simulink model "robotPrototype"  (R2021a)
settings: Solver=ode15s  StartTime=0.0  StopTime=simTime
model workspace: external: MAT-File (data not in the file)
values from neighbouring files (symbols this model uses):
  controlLim = [0.15 3 3]    [simulinkModelParam.mat]
  controlWeight = [0.75 0.6 0.5]    [simulinkModelParam.mat]
  delta = 0.3    [robotParameters.m]    (also in simulinkModelParam.mat = 0.25)
  deltaPlus = 0.20    (= 0.2)    [robotParameters.m]    (also in simulinkModelParam.mat = 0.15)
  den_CoP = [1 -1.84477840502 0.855986791935]    [simulinkModelParam.mat]
  den_zddot = [1 -1.92894226325 0.931381682127]    [simulinkModelParam.mat]
  f_0 = [1,1; deltaPlus-CoM_0(1), -(delta-deltaPlus+CoM_0(1))]\[m*9.81/2;0]    [robotParameters.m]
  f_sample = 500    [robotParameters.m]    (also in simulinkModelParam.mat = 1000)
  filterCoef = 50    [robotParameters.m]    (also in simulinkModelParam.mat = 1000)
  foot_x = delta    (= 0.3)    [robotParameters.m]    (also in simulinkModelParam.mat = 0.25)
  foot_y = delta/3    (= 0.1)    [robotParameters.m]    (also in simulinkModelParam.mat = 0.0833333333333)
  foot_z = 0.03    [robotParameters.m]    (also in simulinkModelParam.mat = 0.02)
  kd_ank = 0    [robotParameters.m]    (also in simulinkModelParam.mat)
  kd_hip = 250    [robotParameters.m]    (also in simulinkModelParam.mat = 12)
  kd_knee1 = 0.02    [robotParameters.m]    (also in simulinkModelParam.mat = 0)
  kd_knee2 = 500    [robotParameters.m]    (also in simulinkModelParam.mat = 150)
  ki_ank = 1800    [robotParameters.m]    (also in simulinkModelParam.mat = 500)
  ki_hip = 0    [robotParameters.m]    (also in simulinkModelParam.mat)
  ki_knee1 = 0    [robotParameters.m]    (also in simulinkModelParam.mat = 0.5)
  ki_knee2 = 0    [robotParameters.m]    (also in simulinkModelParam.mat)
  kp_ank = 375    [robotParameters.m]    (also in simulinkModelParam.mat = 325)
  kp_hip = 500    [robotParameters.m]    (also in simulinkModelParam.mat = 25)
  kp_knee1 = 8    [robotParameters.m]    (also in simulinkModelParam.mat = 3)
  kp_knee2 = 1000    [robotParameters.m]    (also in simulinkModelParam.mat = 300)
  L = 0.94*2*legLength    (= 0.7896)    [robotParameters.m]    (also in simulinkModelParam.mat = 0.72)
  legLength = param(1)    [forwardKin.m]    (also in robotParameters.m = 0.42; simulinkModelParam.mat = 0.4)
  legWidth = 0.08    [robotParameters.m]    (also in simulinkModelParam.mat = 0.05)
  limbThickness = 0.05    [robotParameters.m]    (also in simulinkModelParam.mat = 0.025)
  m = param(3)    [forwardKin.m]    (also in robotParameters.m = 70; simulinkModelParam.mat = 25)
  modelProperties = [25 0.5781 0.72]    [simulinkModelParam.mat]
  N = length(theta)    [robotParameters.m]
  num_CoP = [0.00280209672777 0.00560419345555 0.00280209672777]    [simulinkModelParam.mat]
  num_zddot = [0.000609854718717 0.00121970943743 0.000609854718717]    [simulinkModelParam.mat]
  p = 28    [simulinkModelParam.mat]
  pushDur = 0.1    [compareReducedOrderModels.m]    (also in simulinkModelParam.mat; startUpBalanceRobot.m)
  pushForce = pushForce - 2*pushStep    (= 0)    [compareReducedOrderModels.m]    (also in startUpBalanceRobot.m = 494)
  pushOnset = 0.2    [compareReducedOrderModels.m]    (also in simulinkModelParam.mat; startUpBalanceRobot.m)
  segmentMass = struct('torso',0.681, 'thigh', 0.2, 'shank', 0.09, 'foot', 0.029)    [robotParameters.m]
  stateLim = [0.15 1.57079632679 0.8 0.55 1.622 0.3]    [simulinkModelParam.mat]
  stateWeight = [3 0.5 0.3 9 0.25 0.09]    [simulinkModelParam.mat]
  support_x = 2.5    [robotParameters.m]    (also in simulinkModelParam.mat)
  support_y = 2.5    [robotParameters.m]    (also in simulinkModelParam.mat)
  support_z = 0.1    [robotParameters.m]    (also in simulinkModelParam.mat)
  torsoCoM = param(2)    [forwardKin.m]    (also in robotParameters.m = 0.235; simulinkModelParam.mat = 0.1875)
  torsoLength = 0.47    [robotParameters.m]    (also in simulinkModelParam.mat = 0.25)
  zmax = (2*legLength)*sin(acos(0.2/(2*legLength)))+ankleOffset    [robotParameters.m]    (also in simulinkModelParam.mat = 0.8)
  zmin = 0.6+ ankleOffset    (= 0.67)    [robotParameters.m]    (also in simulinkModelParam.mat = 0.6)
undefined symbols (not defined in the file or in its folder): controlRateWeight, den_qdot, nlobjLIP, num_qdot, X, Y, Z
libraries: sm_lib x27, nesl_utility x19, pid_lib x16, robotmaniplib x16, simulink_extras x16, mpclib x4, Contact_Forces_Lib x4, simulink x2
(part 1 of 3)
settings Model: SimulationMode=accelerator  OrderedModelArguments=off  Creator=tomhu  LastModifiedBy=tomhu
settings SimscapeCC: SimscapeNormalizeSystem=off
settings DiagnosticsConfigSet: SimMechanicsRigidlyBoundBlock=warning
settings ExplorerConfigSet: SimMechanicsOpenEditorOnUpdate=off

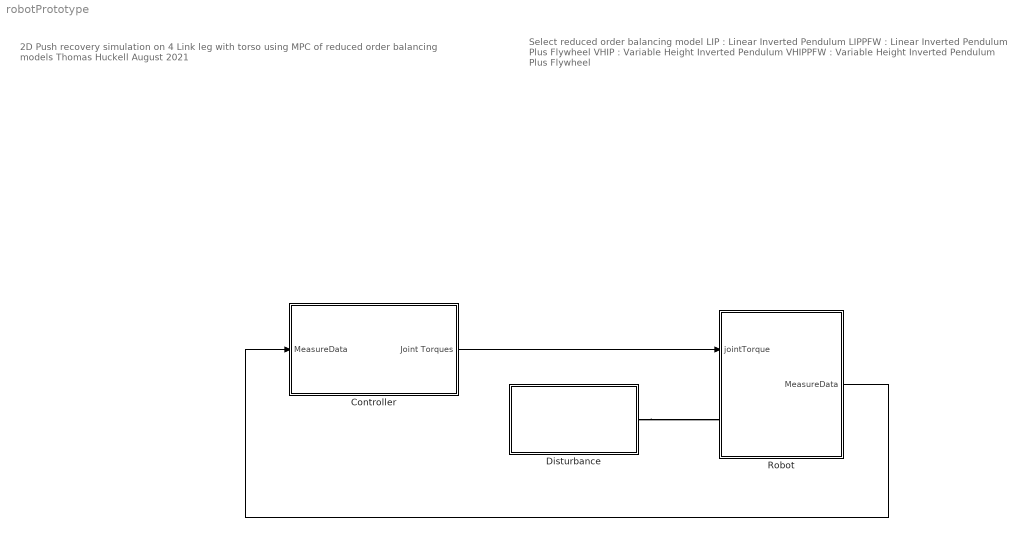
== system robotPrototype ==
  note: Select reduced order balancing model
      | LIP : Linear Inverted Pendulum
      | LIPPFW : Linear Inverted Pendulum Plus Flywheel
      | VHIP : Variable Height Inverted Pendulum
      | VHIPPFW : Variable Height Inverted Pendulum Plus Flywheel
  note: 2D Push recovery simulation on 4 Link leg with torso using MPC of reduced order balancing models
      |
      | Thomas Huckell
      |
      | August 2021
  Controller : Subsystem
  Disturbance : Subsystem  mask{M=pushForce, pushDur=pushDur, Ts=pushOnset}
      mask prompts: M "Push Force [N]"; pushDur "Push Duration [s]"; Ts "Push Onset [s]"
  Robot : Subsystem
      mask Display: image('C:\Users\tomhu\OneDrive - Queen''s University\MASc\Research\Robot\Model\Figures\RobotConfigure.PNG'); % Use "Edit Image" on toolstrip to change.
  wires:
  Controller/1(Joint Torques) -> Robot/1(jointTorque)
  Robot/1(MeasureData) -> Controller/1(MeasureData)
  connections:
  Disturbance/RConn1 -- Robot/LConn1

== system robotPrototype/Controller ==
  MeasureData : Inport
  Bus Creator : BusCreator  Inputs=3
  Bus Selector : BusSelector  OutputSignals=state
  Bus Selector1 : BusSelector  OutputSignals=ankle,knee,hip
  MPC : Subsystem  Variant=on
  Saturation1 : Saturate  UpperLimit=500  LowerLimit=-500  LinearizeAsGain=off
  Saturation2 : Saturate  UpperLimit=500  LowerLimit=-500  LinearizeAsGain=off
  Saturation3 : Saturate  UpperLimit=500  LowerLimit=-500  LinearizeAsGain=off
  To Workspace : ToWorkspace  VariableName=jointTorques  SaveFormat=Timeseries  SampleTime=-1
  To Workspace1 : ToWorkspace  VariableName=mpcControl  SaveFormat=Timeseries  SampleTime=-1
  Variant Subsystem : Subsystem  Variant=on
  Joint Torques : Outport
  wires:
  Bus Selector/1 -> MPC/1(X)  "<state>"
  MeasureData/1 -> Variant Subsystem/2(measureData), Bus Selector/1
  MPC/1(mv) -> To Workspace1/1, Variant Subsystem/1(mv)
  Variant Subsystem/1(jointTorque) -> Bus Selector1/1
  Bus Creator/1 -> To Workspace/1, Joint Torques/1
  Saturation2/1 -> Bus Creator/1  "ankle"
  Saturation1/1 -> Bus Creator/2  "knee"
  Saturation3/1 -> Bus Creator/3  "hip"
  Bus Selector1/1 -> Saturation2/1  "<ankle>"
  Bus Selector1/2 -> Saturation1/1  "<knee>"
  Bus Selector1/3 -> Saturation3/1  "<hip>"

== system robotPrototype/Disturbance ==
  Add : Sum
  External Force and Torque : sm_lib/Forces and Torques/External Force and Torque  ForceResolutionFrame=AttachedFrame  EnableForceX=on  EnableForceY=off  EnableForceZ=off  EnableForce=off  TorqueResolutionFrame=AttachedFrame  EnableTorqueX=off  EnableTorqueY=off  EnableTorqueZ=off  EnableTorque=off
  Simulink-PS Converter4 : nesl_utility/Simulink-PS Converter  PhysicalDomain=network_engine_domain  SubClassName=ps_input  LeftPortType=input  RightPortType=output  PseudoPeriodic=off  Frequencies=[]  NoiseDistribution=none  NoiseParameters=[]  Unit=1  AffineConversion=off  FilteringAndDerivatives=provide  SimscapeFilterOrder=1  InputFilterTimeConstant=0.001  UdotUserProvided=0
      settings: SourceProductBaseCode=PW,SS
  Step : Step  Time=Ts  After=M  SampleTime=0
  Step1 : Step  Time=Ts+pushDur  After=-M  SampleTime=0
  Push Disturbance : PMIOPort  Side=Right
  wires:
  Add/1 -> Simulink-PS Converter4/1
  Step/1 -> Add/1
  Step1/1 -> Add/2
  connections:
  Simulink-PS Converter4/RConn1 -- External Force and Torque/LConn1
  External Force and Torque/RConn1 -- Push Disturbance/RConn1

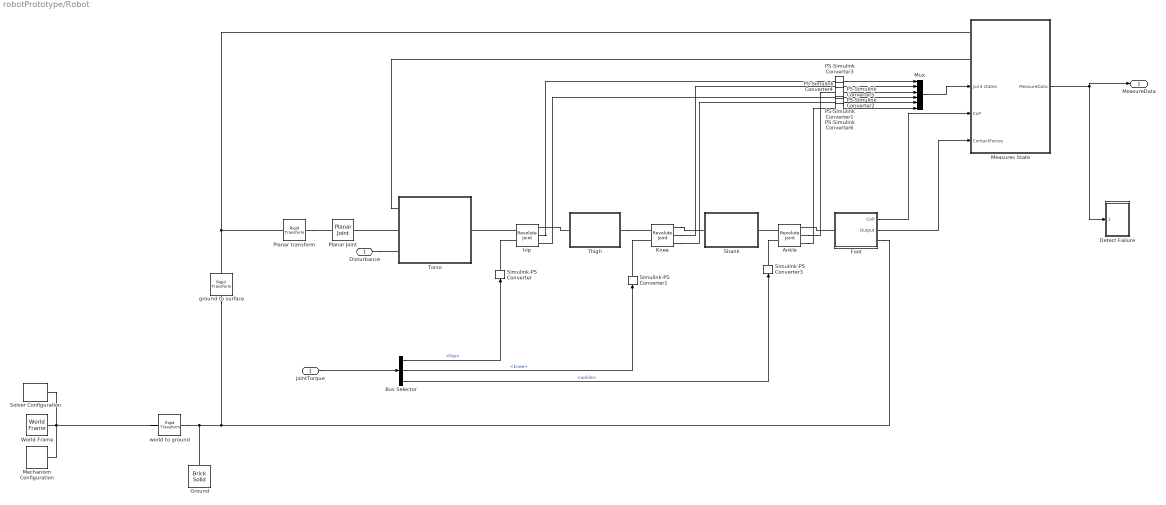
== system robotPrototype/Robot ==
  jointTorque : Inport
  Ankle : sm_lib/Joints/Revolute Joint  JointMode=Normal  SenseConstraintForce=off  SenseConstraintForceX=off  SenseConstraintForceY=off  SenseConstraintForceZ=off  SenseConstraintTorque=off  SenseConstraintTorqueX=off  SenseConstraintTorqueY=off  SenseConstraintTorqueZ=off  SenseTotalForce=off  SenseTotalForceX=off  SenseTotalForceY=off  SenseTotalForceZ=off  SenseTotalTorque=off  SenseTotalTorqueX=off  SenseTotalTorqueY=off  SenseTotalTorqueZ=off  CompositeWrenchDir=FollowerOnBase  CompositeWrenchFrame=BaseFrame  EquilibriumPosition=0  EquilibriumPositionUnits=deg  SpringStiffness=0  SpringStiffnessUnits=N*m/deg  DampingCoefficient=0.001  DampingCoefficientUnits=N*m/(deg/s)  TorqueActuationMode=InputTorque  MotionActuationMode=ComputedMotion  SensePosition=on  SenseVelocity=on  SenseAcceleration=off  SenseTorqueForce=off  SenseLowerLimitTorqueForce=off  SenseUpperLimitTorqueForce=off  LowerLimitSpecify=on  LowerLimitBound=-90  LowerLimitBoundUnits=deg  LowerLimitStiffness=1e4  LowerLimitStiffnessUnits=N*m/deg  LowerLimitDamping=10  LowerLimitDampingUnits=N*m/(deg/s)  LowerLimitTransitionRegionWidth=0.1  LowerLimitTransitionRegionWidthUnits=deg  UpperLimitSpecify=on  UpperLimitBound=90  UpperLimitBoundUnits=deg  UpperLimitStiffness=1e4  UpperLimitStiffnessUnits=N*m/deg  UpperLimitDamping=10  UpperLimitDampingUnits=N*m/(deg/s)  UpperLimitTransitionRegionWidth=0.1  UpperLimitTransitionRegionWidthUnits=deg  PositionTargetSpecify=on  PositionTargetPriority=High  PositionTargetValue=t3_0  PositionTargetValueUnits=rad  VelocityTargetSpecify=off  VelocityTargetPriority=High  VelocityTargetValue=0  VelocityTargetValueUnits=deg/s
  Bus Selector : BusSelector  OutputSignals=hip,knee,ankle
  Detect Failure : Subsystem
  Foot : Subsystem
  Ground : sm_lib/Body Elements/Brick Solid  GraphicAmbientColor=[0.15 0.15 0.15 1.0]  BasedOnType=Density  BrickDimensions=[support_x, support_y, support_z]  BrickDimensionUnits=m  CenterOfMass=[0 0 0]  CenterOfMassUnits=m  GraphicDiffuseColor=[0.0 0.4 0.2]  Density=1000  DensityUnits=kg/m^3  DoExposeReferenceFrame=on  GraphicEmissiveColor=[0.0 0.0 0.0 1.0]  ExportEntireGeometry=off  SerializedFrames=<Frames/>  MarkerShape=Sphere  MarkerSize=10  GraphicType=FromGeometry  InertiaType=CalculateFromGeometry  Mass=1  MassUnits=kg  MomentsOfInertia=[1 1 1]  MomentsOfInertiaUnits=kg*m^2  GraphicOpacity=0.3  ProductsOfInertia=[0 0 0]  ProductsOfInertiaUnits=kg*m^2  GraphicShininess=75  GraphicSpecularColor=[0.5 0.5 0.5 1.0]  GraphicVisPropType=SimpleVisualProperties
  Knee : sm_lib/Joints/Revolute Joint  JointMode=Normal  SenseConstraintForce=off  SenseConstraintForceX=off  SenseConstraintForceY=off  SenseConstraintForceZ=off  SenseConstraintTorque=off  SenseConstraintTorqueX=off  SenseConstraintTorqueY=off  SenseConstraintTorqueZ=off  SenseTotalForce=off  SenseTotalForceX=off  SenseTotalForceY=off  SenseTotalForceZ=off  SenseTotalTorque=off  SenseTotalTorqueX=off  SenseTotalTorqueY=off  SenseTotalTorqueZ=off  CompositeWrenchDir=FollowerOnBase  CompositeWrenchFrame=BaseFrame  EquilibriumPosition=0  EquilibriumPositionUnits=deg  SpringStiffness=0  SpringStiffnessUnits=N*m/deg  DampingCoefficient=0.001  DampingCoefficientUnits=N*m/(deg/s)  TorqueActuationMode=InputTorque  MotionActuationMode=ComputedMotion  SensePosition=on  SenseVelocity=on  SenseAcceleration=off  SenseTorqueForce=off  SenseLowerLimitTorqueForce=off  SenseUpperLimitTorqueForce=off  LowerLimitSpecify=on  LowerLimitBound=-90  LowerLimitBoundUnits=deg  LowerLimitStiffness=1e5  LowerLimitStiffnessUnits=N*m/deg  LowerLimitDamping=10  LowerLimitDampingUnits=N*m/(deg/s)  LowerLimitTransitionRegionWidth=3  LowerLimitTransitionRegionWidthUnits=deg  UpperLimitSpecify=on  UpperLimitBound=0  UpperLimitBoundUnits=deg  UpperLimitStiffness=1e4  UpperLimitStiffnessUnits=N*m/deg  UpperLimitDamping=10  UpperLimitDampingUnits=N*m/(deg/s)  UpperLimitTransitionRegionWidth=2  UpperLimitTransitionRegionWidthUnits=deg  PositionTargetSpecify=on  PositionTargetPriority=High  PositionTargetValue=t2_0  PositionTargetValueUnits=rad  VelocityTargetSpecify=off  VelocityTargetPriority=High  VelocityTargetValue=0  VelocityTargetValueUnits=deg/s
  Measures State : Subsystem
      settings: PortSchema="{\"entries\":[{\"content\":{\"sides\":[{\"content\":{\"connectorIds\":[\"LConn1\",\"LConn2\",\"In1\",\"In2\",\"In3\"]},\"type\":\"ConnectorPlacement.EquallySpacedRectSide\",\"uuid\":\"491601c2-282d-472b-a160-449a44ca8289\"},{\"content\":{\"connectorIds\":[\"Out1\"],\"side\":\"RIGHT\"},\"type\":\"ConnectorPlacement.EquallySpacedRectSide\",\"uuid\":\"5be6c390-8aea-4246-9e11-8b08edaa1b58\"},{\"content\":{\"connectorIds\":[],\"side\":\"TOP\"},\"type\":\"ConnectorPlacement.EquallySpacedRectSide\",\"uuid\":\"78d05e4f-efd7-46b6-ad15-3acf80423762\"}]},\"type\":\"ConnectorPlacement.EquallySpacedConnector\",\"uuid\":\"639014c9-32ba-4b2e-824a-b04e55a10a1e\"}],\"packageUris\":[\"http://schema.mathworks.com/mf0/Connector/R2020b\"],\"version\":\"1.0\"}"
  Mechanism Configuration : sm_lib/Utilities/Mechanism Configuration  UniformGravity=Constant  GravityVector=[0 0 -9.80665]  GravityVectorUnits=m/s^2  GravityUnits=m/s^2  LinearizationDelta=0.001  JointModeTransitionNonlinearIterations=2
  Mux : Mux  Inputs=6
  PS-Simulink Converter1 : nesl_utility/PS-Simulink Converter  PhysicalDomain=network_engine_domain  SubClassName=ps_output  LeftPortType=input  RightPortType=output  PseudoPeriodic=off  Frequencies=[]  Unit=rad/s  AffineConversion=off
      settings: SourceProductBaseCode=PW,SS
  PS-Simulink Converter2 : nesl_utility/PS-Simulink Converter  PhysicalDomain=network_engine_domain  SubClassName=ps_output  LeftPortType=input  RightPortType=output  PseudoPeriodic=off  Frequencies=[]  Unit=rad/s  AffineConversion=off
      settings: SourceProductBaseCode=PW,SS
  PS-Simulink Converter3 : nesl_utility/PS-Simulink Converter  PhysicalDomain=network_engine_domain  SubClassName=ps_output  LeftPortType=input  RightPortType=output  PseudoPeriodic=off  Frequencies=[]  Unit=rad  AffineConversion=off
      settings: SourceProductBaseCode=PW,SS
  PS-Simulink Converter4 : nesl_utility/PS-Simulink Converter  PhysicalDomain=network_engine_domain  SubClassName=ps_output  LeftPortType=input  RightPortType=output  PseudoPeriodic=off  Frequencies=[]  Unit=rad  AffineConversion=off
      settings: SourceProductBaseCode=PW,SS
  PS-Simulink Converter5 : nesl_utility/PS-Simulink Converter  PhysicalDomain=network_engine_domain  SubClassName=ps_output  LeftPortType=input  RightPortType=output  PseudoPeriodic=off  Frequencies=[]  Unit=rad  AffineConversion=off
      settings: SourceProductBaseCode=PW,SS
  PS-Simulink Converter6 : nesl_utility/PS-Simulink Converter  PhysicalDomain=network_engine_domain  SubClassName=ps_output  LeftPortType=input  RightPortType=output  PseudoPeriodic=off  Frequencies=[]  Unit=rad/s  AffineConversion=off
      settings: SourceProductBaseCode=PW,SS
  Planar Joint : sm_lib/Joints/Planar Joint  JointMode=Normal  SenseConstraintForce=off  SenseConstraintForceX=off  SenseConstraintForceY=off  SenseConstraintForceZ=off  SenseConstraintTorque=off  SenseConstraintTorqueX=off  SenseConstraintTorqueY=off  SenseConstraintTorqueZ=off  SenseTotalForce=off  SenseTotalForceX=off  SenseTotalForceY=off  SenseTotalForceZ=off  SenseTotalTorque=off  SenseTotalTorqueX=off  SenseTotalTorqueY=off  SenseTotalTorqueZ=off  CompositeWrenchDir=FollowerOnBase  CompositeWrenchFrame=BaseFrame  PxEquilibriumPosition=0  PxEquilibriumPositionUnits=m  PxSpringStiffness=0  PxSpringStiffnessUnits=N/m  PxDampingCoefficient=0  PxDampingCoefficientUnits=N/(m/s)  PxTorqueActuationMode=NoTorque  PxMotionActuationMode=ComputedMotion  PxSensePosition=off  PxSenseVelocity=off  PxSenseAcceleration=off  PxSenseTorqueForce=off  PxSenseLowerLimitTorqueForce=off  PxSenseUpperLimitTorqueForce=off  PxLowerLimitSpecify=off  PxLowerLimitBound=-1  PxLowerLimitBoundUnits=m  PxLowerLimitStiffness=1e6  PxLowerLimitStiffnessUnits=N/m  PxLowerLimitDamping=1e3  PxLowerLimitDampingUnits=N/(m/s)  PxLowerLimitTransitionRegionWidth=1e-4  PxLowerLimitTransitionRegionWidthUnits=m  PxUpperLimitSpecify=off  PxUpperLimitBound=1  PxUpperLimitBoundUnits=m  PxUpperLimitStiffness=1e6  PxUpperLimitStiffnessUnits=N/m  PxUpperLimitDamping=1e3  PxUpperLimitDampingUnits=N/(m/s)  PxUpperLimitTransitionRegionWidth=1e-4  PxUpperLimitTransitionRegionWidthUnits=m  PxPositionTargetSpecify=off  PxPositionTargetPriority=High  PxPositionTargetValue=0  PxPositionTargetValueUnits=m  PxVelocityTargetSpecify=off  PxVelocityTargetPriority=High  PxVelocityTargetValue=0  PxVelocityTargetValueUnits=m/s  PyEquilibriumPosition=0  PyEquilibriumPositionUnits=m  PySpringStiffness=0  PySpringStiffnessUnits=N/m  PyDampingCoefficient=0  PyDampingCoefficientUnits=N/(m/s)  PyTorqueActuationMode=NoTorque  PyMotionActuationMode=ComputedMotion  PySensePosition=off  PySenseVelocity=off  PySenseAcceleration=off  PySenseTorqueForce=off  PySenseLowerLimitTorqueForce=off  PySenseUpperLimitTorqueForce=off  PyLowerLimitSpecify=off  PyLowerLimitBound=-1  PyLowerLimitBoundUnits=m  PyLowerLimitStiffness=1e6  PyLowerLimitStiffnessUnits=N/m  PyLowerLimitDamping=1e3  PyLowerLimitDampingUnits=N/(m/s)  PyLowerLimitTransitionRegionWidth=1e-4  PyLowerLimitTransitionRegionWidthUnits=m  PyUpperLimitSpecify=off  PyUpperLimitBound=1  PyUpperLimitBoundUnits=m  PyUpperLimitStiffness=1e6  PyUpperLimitStiffnessUnits=N/m  PyUpperLimitDamping=1e3  PyUpperLimitDampingUnits=N/(m/s)  PyUpperLimitTransitionRegionWidth=1e-4  PyUpperLimitTransitionRegionWidthUnits=m  PyPositionTargetSpecify=on  PyPositionTargetPriority=High  PyPositionTargetValue="L+torsoLength -  4.4100e-04"  PyPositionTargetValueUnits=m  PyVelocityTargetSpecify=off  PyVelocityTargetPriority=High  PyVelocityTargetValue=0  PyVelocityTargetValueUnits=m/s  RzEquilibriumPosition=0  RzEquilibriumPositionUnits=deg  RzSpringStiffness=0  RzSpringStiffnessUnits=N*m/deg  RzDampingCoefficient=0  RzDampingCoefficientUnits=N*m/(deg/s)  RzTorqueActuationMode=NoTorque  RzMotionActuationMode=ComputedMotion  RzSensePosition=off  RzSenseVelocity=off  RzSenseAcceleration=off  RzSenseTorqueForce=off  RzSenseLowerLimitTorqueForce=off  RzSenseUpperLimitTorqueForce=off  RzLowerLimitSpecify=off  RzLowerLimitBound=-90  RzLowerLimitBoundUnits=deg  RzLowerLimitStiffness=1e4  RzLowerLimitStiffnessUnits=N*m/deg  RzLowerLimitDamping=10  RzLowerLimitDampingUnits=N*m/(deg/s)  RzLowerLimitTransitionRegionWidth=0.1  RzLowerLimitTransitionRegionWidthUnits=deg  RzUpperLimitSpecify=off  RzUpperLimitBound=90  RzUpperLimitBoundUnits=deg  RzUpperLimitStiffness=1e4  RzUpperLimitStiffnessUnits=N*m/deg  RzUpperLimitDamping=10  RzUpperLimitDampingUnits=N*m/(deg/s)  RzUpperLimitTransitionRegionWidth=0.1  RzUpperLimitTransitionRegionWidthUnits=deg  RzPositionTargetSpecify=off  RzPositionTargetPriority=High  RzPositionTargetValue=0  RzPositionTargetValueUnits=deg  RzVelocityTargetSpecify=off  RzVelocityTargetPriority=High  RzVelocityTargetValue=0  RzVelocityTargetValueUnits=deg/s
  Planer transform : sm_lib/Frames and Transforms/Rigid Transform  TranslationMethod=None  TranslationStandardOffset=0  TranslationLengthUnit=m  TranslationStandardAxis=+Z  TranslationCartesianOffset=[0 0 0]  TranslationROffset=0  TranslationROffsetUnits=m  TranslationZOffset=0  TranslationZOffsetUnits=m  TranslationThetaOffset=0  TranslationThetaOffsetUnits=deg  RotationMethod=StandardAxis  RotationAngleUnits=deg  RotationStandardAxis=+X  RotationAngle=90  RotationArbitraryAxis=[0 0 1]  FollAlignAxisA=+X  BaseAlignAxisA=+Y  FollAlignAxisB=+Y  BaseAlignAxisB=+Z  RotationSequenceAxes=FollowerAxes  RotationSequence=XYX  RotationSequenceAngles=[0 0 0]  RotationSequenceAnglesUnits=deg  RotationMatrix=[1 0 0; 0 1 0; 0 0 1]
  Shank : Subsystem
  Simulink-PS Converter : nesl_utility/Simulink-PS Converter  PhysicalDomain=network_engine_domain  SubClassName=ps_input  LeftPortType=input  RightPortType=output  PseudoPeriodic=off  Frequencies=[]  NoiseDistribution=none  NoiseParameters=[]  Unit=1  AffineConversion=off  FilteringAndDerivatives=provide  SimscapeFilterOrder=1  InputFilterTimeConstant=0.001  UdotUserProvided=0
      settings: SourceProductBaseCode=PW,SS
  Simulink-PS Converter1 : nesl_utility/Simulink-PS Converter  PhysicalDomain=network_engine_domain  SubClassName=ps_input  LeftPortType=input  RightPortType=output  PseudoPeriodic=off  Frequencies=[]  NoiseDistribution=none  NoiseParameters=[]  Unit=1  AffineConversion=off  FilteringAndDerivatives=provide  SimscapeFilterOrder=1  InputFilterTimeConstant=0.001  UdotUserProvided=0
      settings: SourceProductBaseCode=PW,SS
  Simulink-PS Converter3 : nesl_utility/Simulink-PS Converter  PhysicalDomain=network_engine_domain  SubClassName=ps_input  LeftPortType=input  RightPortType=output  PseudoPeriodic=off  Frequencies=[]  NoiseDistribution=none  NoiseParameters=[]  Unit=1  AffineConversion=off  FilteringAndDerivatives=provide  SimscapeFilterOrder=1  InputFilterTimeConstant=0.001  UdotUserProvided=0
      settings: SourceProductBaseCode=PW,SS
  Solver Configuration : nesl_utility/Solver Configuration  PhysicalDomain=network_engine_domain  SubClassName=solver  LeftPortType=input  RightPortType=generic  Tones=[]  Harmonics=[]  SimulateNoise=off  Profile=off  UseLocalSampling=off  EnableSwitchedLinearOptims=on  FrequencyDomain=off  UseCCode=off  RelTol=0.001  AbsTol=1e-06  MinStep=1e-09  ToWorkspace=off  RevertToSquareIcSolve=off  NumHomotopyIterations=100  PhasorMode=off  PhasorModeNumHarmonics=1  DoDC=off  ResidualTolerance=1e-09  UseLocalSolver=off  LocalSolverChoice=NE_TRAPEZOIDAL_ADVANCER  LocalSolverSampleTime=0.001  DoFixedCost=off  MaxNonlinIter=3  MaxModeIter=2  ComputeImpulses=off  ImpulseIterations=2  LinearAlgebra=Sparse  EquationFormulation=NE_TIME_EF  DelaysMemoryBudget=1024  AutomaticFiltering=on  FilteringTimeConstant=0.001  PartitionStorageMethod=AS_NEEDED  PartitionMemoryBudget=1024  PartitionMethod=ROBUST
      settings: SourceProductBaseCode=PW,SS
  Thigh : Subsystem
  Torso : Subsystem
  World Frame : sm_lib/Frames and Transforms/World Frame
  ground to surface : sm_lib/Frames and Transforms/Rigid Transform  TranslationMethod=StandardAxis  TranslationStandardOffset=1/2*support_z  TranslationLengthUnit=m  TranslationStandardAxis=+Z  TranslationCartesianOffset=[0 0 0]  TranslationROffset=0  TranslationROffsetUnits=m  TranslationZOffset=0  TranslationZOffsetUnits=m  TranslationThetaOffset=0  TranslationThetaOffsetUnits=deg  RotationMethod=None  RotationAngleUnits=deg  RotationStandardAxis=+Z  RotationAngle=0.0  RotationArbitraryAxis=[0 0 1]  FollAlignAxisA=+X  BaseAlignAxisA=+Y  FollAlignAxisB=+Y  BaseAlignAxisB=+Z  RotationSequenceAxes=FollowerAxes  RotationSequence=XYX  RotationSequenceAngles=[0 0 0]  RotationSequenceAnglesUnits=deg  RotationMatrix=[1 0 0; 0 1 0; 0 0 1]
  hip : sm_lib/Joints/Revolute Joint  JointMode=Normal  SenseConstraintForce=off  SenseConstraintForceX=off  SenseConstraintForceY=off  SenseConstraintForceZ=off  SenseConstraintTorque=off  SenseConstraintTorqueX=off  SenseConstraintTorqueY=off  SenseConstraintTorqueZ=off  SenseTotalForce=off  SenseTotalForceX=off  SenseTotalForceY=off  SenseTotalForceZ=off  SenseTotalTorque=off  SenseTotalTorqueX=off  SenseTotalTorqueY=off  SenseTotalTorqueZ=off  CompositeWrenchDir=FollowerOnBase  CompositeWrenchFrame=BaseFrame  EquilibriumPosition=0  EquilibriumPositionUnits=deg  SpringStiffness=0  SpringStiffnessUnits=N*m/deg  DampingCoefficient=0.001  DampingCoefficientUnits=N*m/(deg/s)  TorqueActuationMode=InputTorque  MotionActuationMode=ComputedMotion  SensePosition=on  SenseVelocity=on  SenseAcceleration=off  SenseTorqueForce=off  SenseLowerLimitTorqueForce=off  SenseUpperLimitTorqueForce=off  LowerLimitSpecify=on  LowerLimitBound=-120  LowerLimitBoundUnits=deg  LowerLimitStiffness=1e4  LowerLimitStiffnessUnits=N*m/deg  LowerLimitDamping=10  LowerLimitDampingUnits=N*m/(deg/s)  LowerLimitTransitionRegionWidth=5  LowerLimitTransitionRegionWidthUnits=deg  UpperLimitSpecify=on  UpperLimitBound=120  UpperLimitBoundUnits=deg  UpperLimitStiffness=1e4  UpperLimitStiffnessUnits=N*m/deg  UpperLimitDamping=10  UpperLimitDampingUnits=N*m/(deg/s)  UpperLimitTransitionRegionWidth=5  UpperLimitTransitionRegionWidthUnits=deg  PositionTargetSpecify=on  PositionTargetPriority=High  PositionTargetValue=t1_0  PositionTargetValueUnits=rad  VelocityTargetSpecify=off  VelocityTargetPriority=High  VelocityTargetValue=0  VelocityTargetValueUnits=deg/s
  world to ground : sm_lib/Frames and Transforms/Rigid Transform  TranslationMethod=Cartesian  TranslationStandardOffset=0  TranslationLengthUnit=m  TranslationStandardAxis=+Z  TranslationCartesianOffset=[0 0 0]  TranslationROffset=0  TranslationROffsetUnits=m  TranslationZOffset=0  TranslationZOffsetUnits=m  TranslationThetaOffset=0  TranslationThetaOffsetUnits=deg  RotationMethod=None  RotationAngleUnits=deg  RotationStandardAxis=+Z  RotationAngle=0.0  RotationArbitraryAxis=[0 0 1]  FollAlignAxisA=+X  BaseAlignAxisA=+Y  FollAlignAxisB=+Y  BaseAlignAxisB=+Z  RotationSequenceAxes=FollowerAxes  RotationSequence=XYX  RotationSequenceAngles=[0 0 0]  RotationSequenceAnglesUnits=deg  RotationMatrix=[1 0 0; 0 1 0; 0 0 1]
  Disturbance : PMIOPort  Side=Left
  MeasureData : Outport
  wires:
  Mux/1 -> Measures State/1(joint states)
  jointTorque/1 -> Bus Selector/1
  PS-Simulink Converter3/1 -> Mux/1
  PS-Simulink Converter4/1 -> Mux/2
  PS-Simulink Converter5/1 -> Mux/3
  Foot/1(CoP) -> Measures State/2(CoP)
  Measures State/1(MeasureData) -> MeasureData/1, Detect Failure/1(MeasureData)
  Bus Selector/1 -> Simulink-PS Converter/1  "<hip>"
  Bus Selector/2 -> Simulink-PS Converter1/1  "<knee>"
  Bus Selector/3 -> Simulink-PS Converter3/1  "<ankle>"
  PS-Simulink Converter1/1 -> Mux/4
  PS-Simulink Converter2/1 -> Mux/5
  PS-Simulink Converter6/1 -> Mux/6
  Foot/2(Output) -> Measures State/3(ContactForces)
  connections:
  Torso/LConn2 -- Planar Joint/RConn1
  Solver Configuration/RConn1 -- world to ground/LConn1 -- World Frame/RConn1 -- Mechanism Configuration/RConn1
  hip/LConn2 -- Simulink-PS Converter/RConn1
  Foot/LConn1 -- Ankle/RConn1
  Knee/RConn1 -- Shank/LConn1
  Disturbance/RConn1 -- Torso/LConn3
  hip/LConn1 -- Torso/RConn1
  Knee/RConn2 -- PS-Simulink Converter4/LConn1
  Measures State/LConn2 -- Torso/LConn1
  Foot/RConn1 -- ground to surface/LConn1 -- world to ground/RConn1 -- Ground/RConn1
  Thigh/LConn1 -- hip/RConn1
  hip/RConn2 -- PS-Simulink Converter3/LConn1
  ground to surface/RConn1 -- Measures State/LConn1 -- Planer transform/LConn1
  Planer transform/RConn1 -- Planar Joint/LConn1
  Simulink-PS Converter3/RConn1 -- Ankle/LConn2
  Ankle/LConn1 -- Shank/RConn1
  Ankle/RConn2 -- PS-Simulink Converter5/LConn1
  Simulink-PS Converter1/RConn1 -- Knee/LConn2
  Thigh/RConn1 -- Knee/LConn1
  PS-Simulink Converter1/LConn1 -- hip/RConn3
  Knee/RConn3 -- PS-Simulink Converter2/LConn1
  Ankle/RConn3 -- PS-Simulink Converter6/LConn1

== system robotPrototype/Controller/MPC ==
  note: 1) Add Subsystem or Model blocks as valid variant choices.
      | 2) You cannot connect blocks at this level. At simulation, connectivity is automatically
      | determined, based on the active variant and port name matching.
  X : Inport
  LIP : Subsystem  VariantControl=model == 1
  LIPPFW : Subsystem  VariantControl=model == 2
  VHIP : Subsystem  VariantControl=model == 3
  VHIPPFW : Subsystem  VariantControl=model == 4
  mv : Outport

== system robotPrototype/Controller/Variant Subsystem ==
  note: 1) Add Subsystem or Model blocks as valid variant choices.
      | 2) You cannot connect blocks at this level. At simulation, connectivity is automatically
      | determined, based on the active variant and port name matching.
  mv : Inport
  measureData : Inport  Port=2
  LIP : Subsystem  VariantControl=model == 1
  LIPPFW : Subsystem  VariantControl=model == 2
  VHIP : Subsystem  VariantControl=model == 3
  VIPPFW : Subsystem  VariantControl=model == 4
  jointTorque : Outport

== system robotPrototype/Robot/Detect Failure ==
  MeasureData : Inport
  Bus Selector1 : BusSelector  OutputSignals=jointPos
  Bus Selector2 : BusSelector  OutputSignals=X_hip
  Demux : Demux  Outputs=2
  Logical Operator : Logic  Operator=OR  AllPortsSameDT=off  OutDataTypeStr=boolean
  Stop Simulation : Stop
  Terminator : Terminator
  detect fall : simulink/Logic and Bit Operations/Compare To Constant  relop=<  const=zmin - 0.1  OutDataTypeStr=boolean
  detect jump : simulink/Logic and Bit Operations/Compare To Constant  relop=>  const=zmax + 0.1  OutDataTypeStr=boolean
  wires:
  Bus Selector1/1 -> Bus Selector2/1  "<jointPos>"
  Bus Selector2/1 -> Demux/1  "<X_hip>"
  Demux/2 -> detect jump/1, detect fall/1
  Logical Operator/1 -> Stop Simulation/1
  Demux/1 -> Terminator/1
  MeasureData/1 -> Bus Selector1/1
  detect fall/1 -> Logical Operator/1
  detect jump/1 -> Logical Operator/2

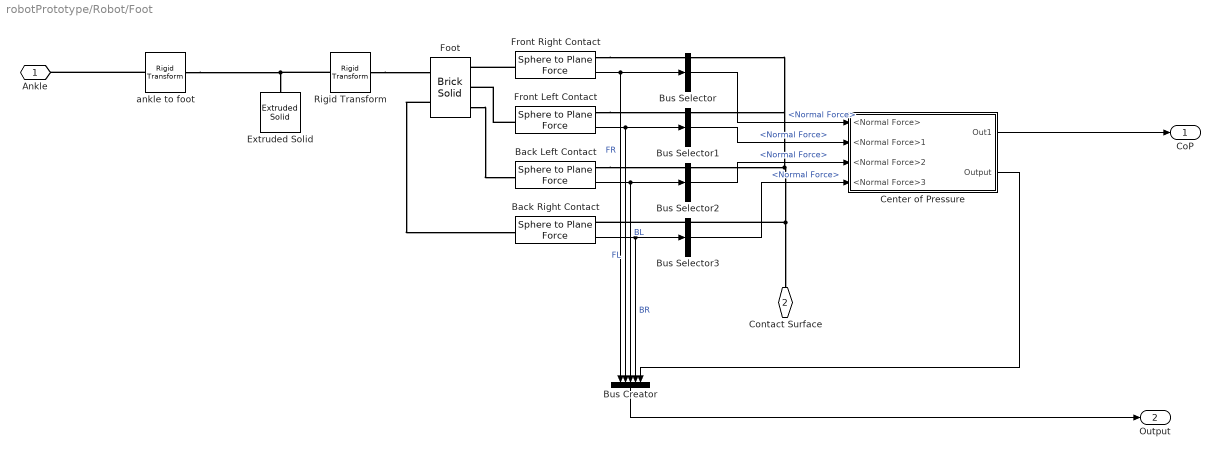
== system robotPrototype/Robot/Foot ==
  Back Left Contact : Contact_Forces_Lib/3D/Sphere to Plane Force  sphere_rad=foot_z/2  plane_lenx=1  plane_leny=1  plane_depth=0.05  force_law=Linear  k_contact=k_contact  b_contact=c_contact  pen_full_damp_F=1e-4  pen_exponent=1  custom_param_1=1  custom_param_2=1  friction_law=Stick-Slip Continuous  mu_kinetic=mu_k  mu_static=mu_s  v_thr=mu_vth  vis_on=off  vis_opc_en=0  vis_len_plaBz=0.005  vis_clr=[0.9 0.2 0.2]  vis_opc=0.7
  Back Right Contact : Contact_Forces_Lib/3D/Sphere to Plane Force  sphere_rad=foot_z/2  plane_lenx=1  plane_leny=1  plane_depth=0.05  force_law=Linear  k_contact=k_contact  b_contact=c_contact  pen_full_damp_F=1e-4  pen_exponent=1  custom_param_1=1  custom_param_2=1  friction_law=Stick-Slip Continuous  mu_kinetic=mu_k  mu_static=mu_s  v_thr=mu_vth  vis_on=off  vis_opc_en=0  vis_len_plaBz=0.005  vis_clr=[0.9 0.2 0.2]  vis_opc=0.7
  Bus Creator : BusCreator  Inputs=5
  Bus Selector{,1..3} (4 alike) : BusSelector  OutputSignals=Normal Force
  Center of Pressure : Subsystem
  Extruded Solid : sm_lib/Body Elements/Extruded Solid  GraphicAmbientColor=[0.15 0.15 0.15 1.0]  BasedOnType=Density  CenterOfMass=[0 0 0]  CenterOfMassUnits=m  GraphicDiffuseColor=[1.0 0.6 0.0]  ExportConvexHullGeometry=off  ExtrusionCrossSection=[0,0; -1/3*delta, -1/2*legWidth; 1/2*delta, - 1/2*legWidth]  ExtrusionCrossSectionUnits=m  Density=1000  DensityUnits=kg/m^3  DoExposeReferenceFrame=on  GraphicEmissiveColor=[0.0 0.0 0.0 1.0]  ExportEntireGeometry=off  ExtrusionLength=1/5* foot_y  ExtrusionLengthUnits=m  ExtrusionType=General  SerializedFrames=<Frames/>  MarkerShape=Sphere  MarkerSize=10  GraphicType=FromGeometry  InertiaType=PointMass  Mass=0.009*m  MassUnits=kg  MomentsOfInertia=[1 1 1]  MomentsOfInertiaUnits=kg*m^2  PolygonNumSides=3  GraphicOpacity=1.0  PolygonOuterRadius=1  PolygonOuterRadiusUnits=m  ProductsOfInertia=[0 0 0]  ProductsOfInertiaUnits=kg*m^2  GraphicShininess=75  GraphicSpecularColor=[0.5 0.5 0.5 1.0]  GraphicVisPropType=SimpleVisualProperties
  Foot : sm_lib/Body Elements/Brick Solid  GraphicAmbientColor=[0.15 0.15 0.15 1.0]  BasedOnType=Mass  BrickDimensions=[foot_x, foot_y, foot_z]  BrickDimensionUnits=m  CenterOfMass=[0 0 0]  CenterOfMassUnits=m  GraphicDiffuseColor=[1.0 0.6 0.0]  Density=1000  DensityUnits=kg/m^3  DoExposeReferenceFrame=on  GraphicEmissiveColor=[0.0 0.0 0.0 1.0]  ExportEntireGeometry=off  SerializedFrames=<Frames><Frame><Id>Frame1</Id><Value><Name>FR</Name><Origin><Source>GeometricFeature</Source><FeatureName>+x -y curve</FeatureName></Origin><PrimaryAxis><DefinedDirection>+Z</DefinedDirection><Source>ReferenceFrame</Source><SourceDirection>+Z</SourceDirection><FeatureName></FeatureName></PrimaryAxis><SecondaryAxis><DefinedDirection>+X</DefinedDirection><Source>ReferenceFrame</Source><SourceDirection>+X</SourceDirection><FeatureName></FeatureName></SecondaryAxis></Value></Frame><Frame><Id>Frame2</Id><Value><Name>FL</Name><Origin><Source>GeometricFeature</Source><FeatureName>+x +y curve</FeatureName></Origin><PrimaryAxis><DefinedDirection>+Z</DefinedDirection><Source>ReferenceFrame</Source><SourceDirection>+Z</SourceDirection><FeatureName></FeatureName></PrimaryAxis><SecondaryAxis><DefinedDirection>+X</DefinedDirection><Source>ReferenceFrame</Source><SourceDirection>+X</SourceDirection><FeatureName></FeatureName></SecondaryAxis></Value></Frame><Frame><Id>Frame3</Id><Value><Name>BR</Name><Origin><Source>GeometricFeature</Source><FeatureName>-x -y curve</FeatureName></Origin><PrimaryAxis><DefinedDirection>+Z</DefinedDirection><Source>ReferenceFrame</Source><SourceDirection>+Z</SourceDirection><FeatureName></FeatureName></PrimaryAxis><SecondaryAxis><DefinedDirection>+X</DefinedDirection><Source>ReferenceFrame</Source><SourceDirection>+X</SourceDirection><FeatureName></FeatureName></SecondaryAxis></Value></Frame><Frame><Id>Frame4</Id><Value><Name>BL</Name><Origin><Source>GeometricFeature</Source><FeatureName>-x +y curve</FeatureName></Origin><PrimaryAxis><DefinedDirection>+Z</DefinedDirection><Source>ReferenceFrame</Source><SourceDirection>+Z</SourceDirection><FeatureName></FeatureName></PrimaryAxis><SecondaryAxis><DefinedDirection>+X</DefinedDirection><Source>ReferenceFrame</Source><SourceDirection>+X</SourceDirection><FeatureName></FeatureName></SecondaryAxis></Value></Frame></Frames>  MarkerShape=Sphere  MarkerSize=10  GraphicType=FromGeometry  InertiaType=CalculateFromGeometry  Mass=.02*m  MassUnits=kg  MomentsOfInertia=[1 1 1]  MomentsOfInertiaUnits=kg*m^2  GraphicOpacity=1.0  ProductsOfInertia=[0 0 0]  ProductsOfInertiaUnits=kg*m^2  GraphicShininess=75  GraphicSpecularColor=[0.5 0.5 0.5 1.0]  GraphicVisPropType=SimpleVisualProperties
  Front Left Contact : Contact_Forces_Lib/3D/Sphere to Plane Force  sphere_rad=foot_z/2  plane_lenx=1  plane_leny=1  plane_depth=0.05  force_law=Linear  k_contact=k_contact  b_contact=c_contact  pen_full_damp_F=1e-4  pen_exponent=1  custom_param_1=1  custom_param_2=1  friction_law=Stick-Slip Continuous  mu_kinetic=mu_k  mu_static=mu_s  v_thr=mu_vth  vis_on=off  vis_opc_en=0  vis_len_plaBz=0.005  vis_clr=[0.9 0.2 0.2]  vis_opc=0.7
  Front Right Contact : Contact_Forces_Lib/3D/Sphere to Plane Force  sphere_rad=foot_z/2  plane_lenx=1  plane_leny=1  plane_depth=0.05  force_law=Linear  k_contact=k_contact  b_contact=c_contact  pen_full_damp_F=1e-4  pen_exponent=1  custom_param_1=1  custom_param_2=1  friction_law=Stick-Slip Continuous  mu_kinetic=mu_k  mu_static=mu_s  v_thr=mu_vth  vis_on=off  vis_opc_en=0  vis_len_plaBz=0.005  vis_clr=[0.9 0.2 0.2]  vis_opc=0.7
  Rigid Transform : sm_lib/Frames and Transforms/Rigid Transform  TranslationMethod=Cartesian  TranslationStandardOffset=0  TranslationLengthUnit=m  TranslationStandardAxis=+Z  TranslationCartesianOffset=[deltaPlus-delta/2, -(1/2*(legWidth+foot_z)), 0]  TranslationROffset=0  TranslationROffsetUnits=m  TranslationZOffset=0  TranslationZOffsetUnits=m  TranslationThetaOffset=0  TranslationThetaOffsetUnits=deg  RotationMethod=StandardAxis  RotationAngleUnits=deg  RotationStandardAxis=+X  RotationAngle=90  RotationArbitraryAxis=[0 0 1]  FollAlignAxisA=+X  BaseAlignAxisA=+Y  FollAlignAxisB=+Y  BaseAlignAxisB=+Z  RotationSequenceAxes=FollowerAxes  RotationSequence=XYX  RotationSequenceAngles=[0 0 0]  RotationSequenceAnglesUnits=deg  RotationMatrix=[1 0 0; 0 1 0; 0 0 1]
  ankle to foot : sm_lib/Frames and Transforms/Rigid Transform  TranslationMethod=None  TranslationStandardOffset=0  TranslationLengthUnit=m  TranslationStandardAxis=+Z  TranslationCartesianOffset=[0 0 0]  TranslationROffset=0  TranslationROffsetUnits=m  TranslationZOffset=0  TranslationZOffsetUnits=m  TranslationThetaOffset=0  TranslationThetaOffsetUnits=deg  RotationMethod=None  RotationAngleUnits=deg  RotationStandardAxis=+Y  RotationAngle=180  RotationArbitraryAxis=[0 0 1]  FollAlignAxisA=+X  BaseAlignAxisA=+Y  FollAlignAxisB=+Y  BaseAlignAxisB=+Z  RotationSequenceAxes=FollowerAxes  RotationSequence=XYX  RotationSequenceAngles=[0 0 0]  RotationSequenceAnglesUnits=deg  RotationMatrix=[1 0 0; 0 1 0; 0 0 1]
  Ankle : PMIOPort  Side=Left
  Contact Surface : PMIOPort  Port=2  Side=Right
  CoP : Outport
  Output : Outport  Port=2
  wires:
  Bus Selector1/1 -> Center of Pressure/2(<Normal Force>1)  "<Normal Force>"
  Front Right Contact/1 -> Bus Selector/1, Bus Creator/1  "FR"
  Center of Pressure/1(Out1) -> CoP/1
  Front Left Contact/1 -> Bus Selector1/1, Bus Creator/2  "FL"
  Back Right Contact/1 -> Bus Selector3/1, Bus Creator/4  "BR"
  Back Left Contact/1 -> Bus Selector2/1, Bus Creator/3  "BL"
  Bus Selector/1 -> Center of Pressure/1(<Normal Force>)  "<Normal Force>"
  Bus Selector3/1 -> Center of Pressure/4(<Normal Force>3)  "<Normal Force>"
  Bus Selector2/1 -> Center of Pressure/3(<Normal Force>2)  "<Normal Force>"
  Bus Creator/1 -> Output/1
  Center of Pressure/2(Output) -> Bus Creator/5
  connections:
  Rigid Transform/RConn1 -- Foot/RConn1
  Front Left Contact/LConn1 -- Foot/LConn2
  ankle to foot/RConn1 -- Rigid Transform/LConn1 -- Extruded Solid/RConn1
  Back Left Contact/RConn1 -- Back Right Contact/RConn1 -- Contact Surface/RConn1 -- Front Right Contact/RConn1 -- Front Left Contact/RConn1
  Foot/LConn3 -- Back Left Contact/LConn1
  Foot/RConn2 -- Back Right Contact/LConn1
  Front Right Contact/LConn1 -- Foot/LConn1
  ankle to foot/LConn1 -- Ankle/RConn1

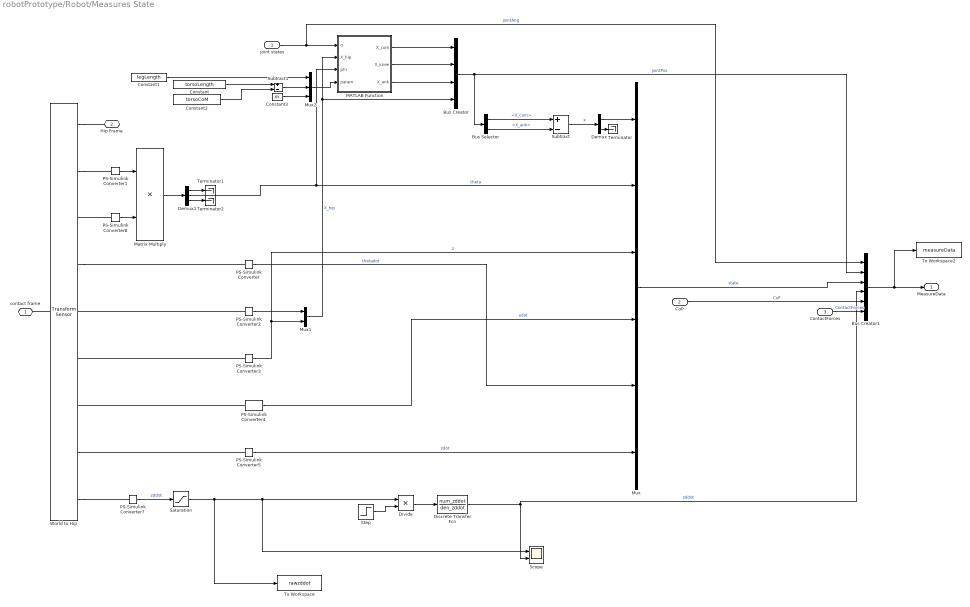
== system robotPrototype/Robot/Measures State ==
  joint states : Inport
  CoP : Inport  Port=2
  ContactForces : Inport  Port=3
  Bus Creator : BusCreator  Inputs=4
  Bus Creator1 : BusCreator  Inputs=6
  Bus Selector : BusSelector  OutputSignals=X_com,X_ank
  Constant : Constant  Value=torsoLength
  Constant1 : Constant  Value=legLength
  Constant2 : Constant  Value=torsoCoM
  Constant3 : Constant  Value=m
  Demux : Demux  Outputs=2
  Demux1 : Demux  Outputs=3
  Discrete Transfer Fcn : DiscreteTransferFcn  Numerator=num_zddot  Denominator=den_zddot  SampleTime=1/f_sample
  Divide : Product  Inputs=**
  MATLAB Function : MATLAB Function  TreatAsAtomicUnit=on
  Matrix Multiply : Product
  Mux : Mux  Inputs=6
  Mux1 : Mux  Inputs=2
  Mux2 : Mux  Inputs=3
  PS-Simulink Converter : nesl_utility/PS-Simulink Converter  PhysicalDomain=network_engine_domain  SubClassName=ps_output  LeftPortType=input  RightPortType=output  PseudoPeriodic=off  Frequencies=[]  Unit=inherit  AffineConversion=off
      settings: SourceProductBaseCode=PW,SS
  PS-Simulink Converter1 : nesl_utility/PS-Simulink Converter  PhysicalDomain=network_engine_domain  SubClassName=ps_output  LeftPortType=input  RightPortType=output  PseudoPeriodic=off  Frequencies=[]  Unit=rad  AffineConversion=off
      settings: SourceProductBaseCode=PW,SS
  PS-Simulink Converter2 : nesl_utility/PS-Simulink Converter  PhysicalDomain=network_engine_domain  SubClassName=ps_output  LeftPortType=input  RightPortType=output  PseudoPeriodic=off  Frequencies=[]  Unit=m  AffineConversion=off
      settings: SourceProductBaseCode=PW,SS
  PS-Simulink Converter3 : nesl_utility/PS-Simulink Converter  PhysicalDomain=network_engine_domain  SubClassName=ps_output  LeftPortType=input  RightPortType=output  PseudoPeriodic=off  Frequencies=[]  Unit=m  AffineConversion=off
      settings: SourceProductBaseCode=PW,SS
  PS-Simulink Converter4 : nesl_utility/PS-Simulink Converter  PhysicalDomain=network_engine_domain  SubClassName=ps_output  LeftPortType=input  RightPortType=output  PseudoPeriodic=off  Frequencies=[]  Unit=m/s  AffineConversion=off
      settings: SourceProductBaseCode=PW,SS
  PS-Simulink Converter5 : nesl_utility/PS-Simulink Converter  PhysicalDomain=network_engine_domain  SubClassName=ps_output  LeftPortType=input  RightPortType=output  PseudoPeriodic=off  Frequencies=[]  Unit=m/s  AffineConversion=off
      settings: SourceProductBaseCode=PW,SS
  PS-Simulink Converter7 : nesl_utility/PS-Simulink Converter  PhysicalDomain=network_engine_domain  SubClassName=ps_output  LeftPortType=input  RightPortType=output  PseudoPeriodic=off  Frequencies=[]  Unit=inherit  AffineConversion=off
      settings: SourceProductBaseCode=PW,SS
  PS-Simulink Converter8 : nesl_utility/PS-Simulink Converter  PhysicalDomain=network_engine_domain  SubClassName=ps_output  LeftPortType=input  RightPortType=output  PseudoPeriodic=off  Frequencies=[]  Unit=inherit  AffineConversion=off
      settings: SourceProductBaseCode=PW,SS
  Saturation : Saturate  UpperLimit=9.81  LowerLimit=-9.81
  Scope : Scope  NumInputPorts=2
  Step : Step  Time=0.2  SampleTime=0
  Subtract : Sum  Inputs=+-
  Subtract1 : Sum  Inputs=+-
  Terminator : Terminator
  Terminator1 : Terminator
  Terminator2 : Terminator
  To Workspace : ToWorkspace  VariableName=rawzddot  SaveFormat=Timeseries  SampleTime=1/f_sample
  To Workspace2 : ToWorkspace  VariableName=measureData  SaveFormat=Timeseries  SampleTime=-1
  World to Hip : sm_lib/Frames and Transforms/Transform Sensor  MeasurementFrame=World  SenseAngle=on  SenseAxis=on  SenseAngle1=off  SenseAngle2=off  SenseAngle3=off  SenseQ=off  SenseR=off  SenseOmegaX=off  SenseOmegaY=on  SenseOmegaZ=off  SenseOmega1=off  SenseOmega2=off  SenseOmega3=off  SenseQDot=off  SenseRDot=off  SenseAlphaX=off  SenseAlphaY=off  SenseAlphaZ=off  SenseAlpha1=off  SenseAlpha2=off  SenseAlpha3=off  SenseQDDot=off  SenseRDDot=off  SenseX=on  SenseY=off  SenseZ=on  SenseRad=off  SenseAzim=off  SenseDist=off  SenseInc=off  SenseXDot=on  SenseYDot=off  SenseZDot=on  SenseRadDot=off  SenseAzimDot=off  SenseDistDot=off  SenseIncDot=off  SenseXDDot=off  SenseYDDot=off  SenseZDDot=on  SenseRadDDot=off  SenseAzimDDot=off  SenseDistDDot=off  SenseIncDDot=off
  contact frame : PMIOPort  Side=Left
  Hip Frame : PMIOPort  Port=2  Side=Left
  MeasureData : Outport
  wires:
  PS-Simulink Converter3/1 -> Mux1/2, Mux/3  "z"
  PS-Simulink Converter5/1 -> Mux/6  "zdot"
  PS-Simulink Converter4/1 -> Mux/4  "xdot"
  PS-Simulink Converter2/1 -> Mux1/1
  joint states/1 -> Bus Creator1/1, MATLAB Function/1(q)  "jointAng"
  Mux1/1 -> MATLAB Function/2(X_hip), Bus Creator/4  "X_hip"
  MATLAB Function/1(X_com) -> Bus Creator/1
  PS-Simulink Converter8/1 -> Matrix Multiply/2
  PS-Simulink Converter1/1 -> Matrix Multiply/1
  Matrix Multiply/1 -> Demux1/1
  Demux1/1 -> Terminator1/1
  Demux1/3 -> Terminator2/1
  Demux1/2 -> Mux/2, MATLAB Function/3(phi)  "theta"
  PS-Simulink Converter/1 -> Mux/5  "thetadot"
  MATLAB Function/2(X_knee) -> Bus Creator/2
  MATLAB Function/3(X_ank) -> Bus Creator/3
  Subtract/1 -> Demux/1  "x"
  Constant1/1 -> Mux2/1
  Mux2/1 -> MATLAB Function/4(param)
  Bus Creator/1 -> Bus Creator1/2, Bus Selector/1  "jointPos"
  Constant/1 -> Subtract1/1
  Constant2/1 -> Subtract1/2
  Subtract1/1 -> Mux2/2
  Demux/1 -> Mux/1
  Bus Selector/2 -> Subtract/2  "<X_ank>"
  Mux/1 -> Bus Creator1/3  "state"
  Bus Creator1/1 -> MeasureData/1, To Workspace2/1
  CoP/1 -> Bus Creator1/5  "CoP"
  Saturation/1 -> To Workspace/1, Divide/1, Scope/1
  Demux/2 -> Terminator/1
  PS-Simulink Converter7/1 -> Saturation/1  "zddot"
  Constant3/1 -> Mux2/3
  Bus Selector/1 -> Subtract/1  "<X_com>"
  Step/1 -> Divide/2
  Discrete Transfer Fcn/1 -> Scope/2, Bus Creator1/4  "zddot"
  Divide/1 -> Discrete Transfer Fcn/1
  ContactForces/1 -> Bus Creator1/6  "ContactForces"
  connections:
  World to Hip/LConn1 -- contact frame/RConn1
  World to Hip/RConn1 -- Hip Frame/RConn1
  World to Hip/RConn9 -- PS-Simulink Converter7/LConn1
  PS-Simulink Converter5/LConn1 -- World to Hip/RConn8
  PS-Simulink Converter4/LConn1 -- World to Hip/RConn7
  PS-Simulink Converter3/LConn1 -- World to Hip/RConn6
  PS-Simulink Converter2/LConn1 -- World to Hip/RConn5
  World to Hip/RConn2 -- PS-Simulink Converter1/LConn1
  PS-Simulink Converter8/LConn1 -- World to Hip/RConn3
  World to Hip/RConn4 -- PS-Simulink Converter/LConn1

== system robotPrototype/Robot/Shank ==
  Shank : sm_lib/Body Elements/Extruded Solid  GraphicAmbientColor=[0.15 0.15 0.15 1.0]  BasedOnType=Mass  CenterOfMass=[0 0 0]  CenterOfMassUnits=m  GraphicDiffuseColor=[1.0 1.0 0.0]  ExportConvexHullGeometry=off  ExtrusionCrossSection=shank_xy  ExtrusionCrossSectionUnits=m  Density=1000  DensityUnits=kg/m^3  DoExposeReferenceFrame=on  GraphicEmissiveColor=[0.0 0.0 0.0 1.0]  ExportEntireGeometry=off  ExtrusionLength=limbThickness  ExtrusionLengthUnits=m  ExtrusionType=General  SerializedFrames=<Frames/>  MarkerShape=Sphere  MarkerSize=10  GraphicType=FromGeometry  InertiaType=CalculateFromGeometry  Mass=segmentMass.shank*m  MassUnits=kg  MomentsOfInertia=[1 1 1]  MomentsOfInertiaUnits=kg*m^2  PolygonNumSides=3  GraphicOpacity=1.0  PolygonOuterRadius=1  PolygonOuterRadiusUnits=m  ProductsOfInertia=[0 0 0]  ProductsOfInertiaUnits=kg*m^2  GraphicShininess=75  GraphicSpecularColor=[0.5 0.5 0.5 1.0]  GraphicVisPropType=SimpleVisualProperties
  knee to shank : sm_lib/Frames and Transforms/Rigid Transform  TranslationMethod=None  TranslationStandardOffset=0  TranslationLengthUnit=m  TranslationStandardAxis=+Z  TranslationCartesianOffset=[0 0 0]  TranslationROffset=0  TranslationROffsetUnits=m  TranslationZOffset=0  TranslationZOffsetUnits=m  TranslationThetaOffset=0  TranslationThetaOffsetUnits=deg  RotationMethod=None  RotationAngleUnits=deg  RotationStandardAxis=+Z  RotationAngle=0.0  RotationArbitraryAxis=[0 0 1]  FollAlignAxisA=+X  BaseAlignAxisA=+Y  FollAlignAxisB=+Y  BaseAlignAxisB=+Z  RotationSequenceAxes=FollowerAxes  RotationSequence=XYX  RotationSequenceAngles=[0 0 0]  RotationSequenceAnglesUnits=deg  RotationMatrix=[1 0 0; 0 1 0; 0 0 1]
  shank to ankle : sm_lib/Frames and Transforms/Rigid Transform  TranslationMethod=StandardAxis  TranslationStandardOffset=legLength  TranslationLengthUnit=m  TranslationStandardAxis=-Y  TranslationCartesianOffset=[0 0 0]  TranslationROffset=0  TranslationROffsetUnits=m  TranslationZOffset=0  TranslationZOffsetUnits=m  TranslationThetaOffset=0  TranslationThetaOffsetUnits=deg  RotationMethod=None  RotationAngleUnits=deg  RotationStandardAxis=+Z  RotationAngle=0.0  RotationArbitraryAxis=[0 0 1]  FollAlignAxisA=+X  BaseAlignAxisA=+Y  FollAlignAxisB=+Y  BaseAlignAxisB=+Z  RotationSequenceAxes=FollowerAxes  RotationSequence=XYX  RotationSequenceAngles=[0 0 0]  RotationSequenceAnglesUnits=deg  RotationMatrix=[1 0 0; 0 1 0; 0 0 1]
  knee : PMIOPort  Side=Left
  ankle : PMIOPort  Port=2  Side=Right
  connections:
  knee to shank/RConn1 -- shank to ankle/LConn1 -- Shank/RConn1
  knee/RConn1 -- knee to shank/LConn1
  shank to ankle/RConn1 -- ankle/RConn1

== system robotPrototype/Robot/Thigh ==
  Thigh : sm_lib/Body Elements/Extruded Solid  GraphicAmbientColor=[0.15 0.15 0.15 1.0]  BasedOnType=Mass  CenterOfMass=[0 0 0]  CenterOfMassUnits=m  GraphicDiffuseColor=[1.0 0.0 0.0]  ExportConvexHullGeometry=off  ExtrusionCrossSection=thigh_xy  ExtrusionCrossSectionUnits=m  Density=1000  DensityUnits=kg/m^3  DoExposeReferenceFrame=on  GraphicEmissiveColor=[0.0 0.0 0.0 1.0]  ExportEntireGeometry=off  ExtrusionLength=limbThickness+0.01  ExtrusionLengthUnits=m  ExtrusionType=General  SerializedFrames=<Frames/>  MarkerShape=Sphere  MarkerSize=10  GraphicType=FromGeometry  InertiaType=CalculateFromGeometry  Mass=segmentMass.thigh*m  MassUnits=kg  MomentsOfInertia=[1 1 1]  MomentsOfInertiaUnits=kg*m^2  PolygonNumSides=3  GraphicOpacity=1.0  PolygonOuterRadius=1  PolygonOuterRadiusUnits=m  ProductsOfInertia=[0 0 0]  ProductsOfInertiaUnits=kg*m^2  GraphicShininess=75  GraphicSpecularColor=[0.5 0.5 0.5 1.0]  GraphicVisPropType=SimpleVisualProperties
  hip to thigh : sm_lib/Frames and Transforms/Rigid Transform  TranslationMethod=None  TranslationStandardOffset=0  TranslationLengthUnit=m  TranslationStandardAxis=+Z  TranslationCartesianOffset=[0 0 0]  TranslationROffset=0  TranslationROffsetUnits=m  TranslationZOffset=0  TranslationZOffsetUnits=m  TranslationThetaOffset=0  TranslationThetaOffsetUnits=deg  RotationMethod=None  RotationAngleUnits=deg  RotationStandardAxis=+Z  RotationAngle=0.0  RotationArbitraryAxis=[0 0 1]  FollAlignAxisA=+X  BaseAlignAxisA=+Y  FollAlignAxisB=+Y  BaseAlignAxisB=+Z  RotationSequenceAxes=FollowerAxes  RotationSequence=XYX  RotationSequenceAngles=[0 0 0]  RotationSequenceAnglesUnits=deg  RotationMatrix=[1 0 0; 0 1 0; 0 0 1]
  thigh to knee : sm_lib/Frames and Transforms/Rigid Transform  TranslationMethod=StandardAxis  TranslationStandardOffset=legLength  TranslationLengthUnit=m  TranslationStandardAxis=-Y  TranslationCartesianOffset=[0 0 0]  TranslationROffset=0  TranslationROffsetUnits=m  TranslationZOffset=0  TranslationZOffsetUnits=m  TranslationThetaOffset=0  TranslationThetaOffsetUnits=deg  RotationMethod=None  RotationAngleUnits=deg  RotationStandardAxis=+Z  RotationAngle=0.0  RotationArbitraryAxis=[0 0 1]  FollAlignAxisA=+X  BaseAlignAxisA=+Y  FollAlignAxisB=+Y  BaseAlignAxisB=+Z  RotationSequenceAxes=FollowerAxes  RotationSequence=XYX  RotationSequenceAngles=[0 0 0]  RotationSequenceAnglesUnits=deg  RotationMatrix=[1 0 0; 0 1 0; 0 0 1]
  Hip : PMIOPort  Side=Left
  Knee : PMIOPort  Port=2  Side=Right
  connections:
  Thigh/RConn1 -- thigh to knee/LConn1 -- hip to thigh/RConn1
  hip to thigh/LConn1 -- Hip/RConn1
  thigh to knee/RConn1 -- Knee/RConn1
